simulink library "VIS_TMS_LIB"  (Simulink 8.8)
settings: Solver=VariableStepAuto  StartTime=0.0  StopTime=10.0  RelTol=1e-3  EnableMultiTasking=on
libraries: cdsEpicsOut x50, cdsFilt x39, cdsFiltCtrl x26, cdsTP x24, cdsEpicsIn x15, cdsRms x12, cdsMuxMatrix x6, cdsEpicsStringIn x6, cdsBit2Word x4, cdsEpicsBinIn x4, cdsWord2Bit x2, VIS_LIB x2
(part 1 of 7)
settings Model: SuppressorTable=22 serialization::archive 11 0 3 0 0 0 11 0  Creator=controls  LastModifiedBy=controls

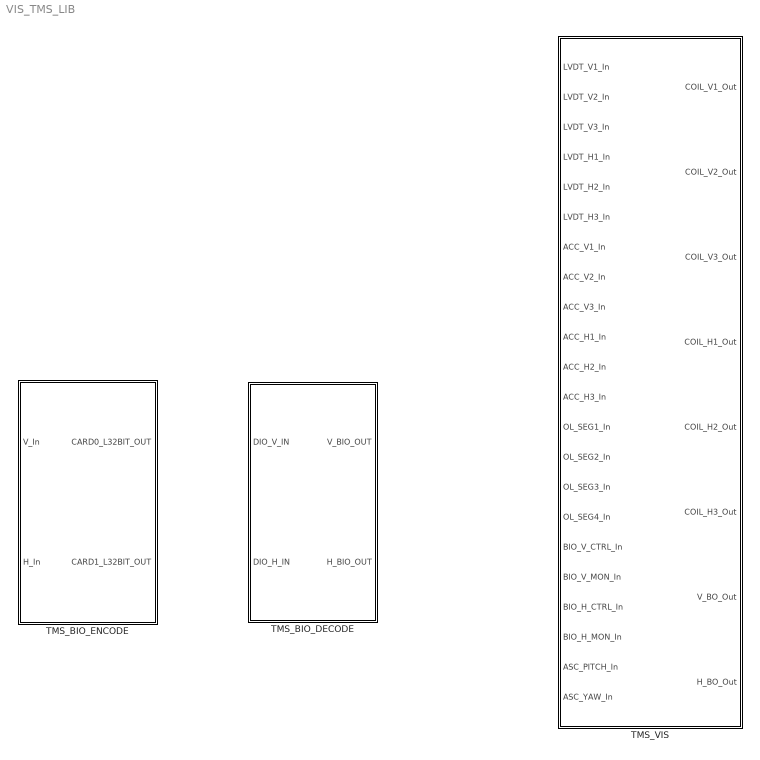
== system VIS_TMS_LIB ==
  TMS_BIO_DECODE : Subsystem
  TMS_BIO_ENCODE : Subsystem
  TMS_VIS : Subsystem

== system VIS_TMS_LIB/TMS_BIO_DECODE ==
  DIO_V_IN : Inport
  DIO_H_IN : Inport  Port=2
  BI1_MON : cdsEpicsOut/Subsystem  Tag=cdsEpicsOutput  Description=|
      | Purpose:                                          
      | Output a FE signal to an EPICS channel.           
      |                                                   
      | Operation:                                        
      | Takes input value and passes it to EPICS record.  
      |                                                   
      | Usage:                                            
      | Name the part with the desired EPICS rrecord name.
      settings: AttributesFormatString=%<Tag>
  BI2_MON : cdsEpicsOut/Subsystem  Tag=cdsEpicsOutput  Description=|
      | Purpose:                                          
      | Output a FE signal to an EPICS channel.           
      |                                                   
      | Operation:                                        
      | Takes input value and passes it to EPICS record.  
      |                                                   
      | Usage:                                            
      | Name the part with the desired EPICS rrecord name.
      settings: AttributesFormatString=%<Tag>
  V_BIO_OUT : Outport
  H_BIO_OUT : Outport  Port=2
  wires:
  DIO_H_IN/1 -> BI2_MON/1
  DIO_V_IN/1 -> BI1_MON/1
  BI1_MON/1 -> V_BIO_OUT/1
  BI2_MON/1 -> H_BIO_OUT/1

== system VIS_TMS_LIB/TMS_BIO_ENCODE ==
  V_In : Inport
  H_In : Inport  Port=2
  BIT2WORD2 : Subsystem
  BIT2WORD3 : Subsystem
  DIO_0_OUT : cdsEpicsOut/Subsystem  Tag=cdsEpicsOutput  Description=|
      | Purpose:                                          
      | Output a FE signal to an EPICS channel.           
      |                                                   
      | Operation:                                        
      | Takes input value and passes it to EPICS record.  
      |                                                   
      | Usage:                                            
      | Name the part with the desired EPICS rrecord name.
      settings: AttributesFormatString=%<Tag>
  DIO_1_OUT : cdsEpicsOut/Subsystem  Tag=cdsEpicsOutput  Description=|
      | Purpose:                                          
      | Output a FE signal to an EPICS channel.           
      |                                                   
      | Operation:                                        
      | Takes input value and passes it to EPICS record.  
      |                                                   
      | Usage:                                            
      | Name the part with the desired EPICS rrecord name.
      settings: AttributesFormatString=%<Tag>
  Ground{2,26,66..67} (4 alike) : Ground
  H_WD_RSET : cdsEpicsBinIn/Subsystem  Tag=cdsEpicsBinIn  Description=|
      | Purpose:                                                                            
      | Create an EPICS binary (0 or 1) input channel to the FE realtime controls.          
      |                                                                                     
      | Operation:                                                                          
      | Outputs value from an EPICS ai record. Value is binary input (bi Epics record type).
      |                                                                                     
      | Usage:                                                                              
      | Name the part with the desired EPICS channel name.
      settings: AttributesFormatString=%<Tag>
  V_WD_RSET : cdsEpicsBinIn/Subsystem  Tag=cdsEpicsBinIn  Description=|
      | Purpose:                                                                            
      | Create an EPICS binary (0 or 1) input channel to the FE realtime controls.          
      |                                                                                     
      | Operation:                                                                          
      | Outputs value from an EPICS ai record. Value is binary input (bi Epics record type).
      |                                                                                     
      | Usage:                                                                              
      | Name the part with the desired EPICS channel name.
      settings: AttributesFormatString=%<Tag>
  cdsWord2Bit : cdsWord2Bit/cdsWord2Bit  Tag=cdsWord2Bit  Description=Generate 16 0/1 outputs from single 16-bit integer input
      settings: AttributesFormatString=cdsWord2Bit
  cdsWord2Bit1 : cdsWord2Bit/cdsWord2Bit  Tag=cdsWord2Bit  Description=Generate 16 0/1 outputs from single 16-bit integer input
      settings: AttributesFormatString=cdsWord2Bit
  CARD0_L32BIT_OUT : Outport
  CARD1_L32BIT_OUT : Outport  Port=2
  wires:
  Ground2/1 -> BIT2WORD2/20(In20), BIT2WORD2/18(In18), BIT2WORD2/19(In19), BIT2WORD2/21(In21), BIT2WORD2/22(In22), BIT2WORD2/23(In23), BIT2WORD2/24(In24), BIT2WORD2/25(In25), BIT2WORD2/26(In26), BIT2WORD2/28(In28), BIT2WORD2/31(In31), BIT2WORD2/32(In32), BIT2WORD2/30(In30), BIT2WORD2/29(In29), BIT2WORD2/27(In27)
  V_In/1 -> cdsWord2Bit/1
  cdsWord2Bit/4 -> BIT2WORD2/4(In4)
  cdsWord2Bit/5 -> BIT2WORD2/5(In5)
  cdsWord2Bit/3 -> BIT2WORD2/3(In3)
  cdsWord2Bit/2 -> BIT2WORD2/2(In2)
  cdsWord2Bit/6 -> BIT2WORD2/6(In6)
  cdsWord2Bit/1 -> BIT2WORD2/1(In1)
  cdsWord2Bit/7 -> BIT2WORD2/7(In7)
  cdsWord2Bit/8 -> BIT2WORD2/8(In8)
  cdsWord2Bit/9 -> BIT2WORD2/9(In9)
  cdsWord2Bit/10 -> BIT2WORD2/10(In10)
  cdsWord2Bit/11 -> BIT2WORD2/11(In11)
  Ground26/1 -> BIT2WORD3/20(In20), BIT2WORD3/18(In18), BIT2WORD3/19(In19), BIT2WORD3/21(In21), BIT2WORD3/22(In22), BIT2WORD3/23(In23), BIT2WORD3/24(In24), BIT2WORD3/25(In25), BIT2WORD3/26(In26), BIT2WORD3/28(In28), BIT2WORD3/31(In31), BIT2WORD3/32(In32), BIT2WORD3/30(In30), BIT2WORD3/29(In29), BIT2WORD3/27(In27)
  H_In/1 -> cdsWord2Bit1/1
  cdsWord2Bit1/4 -> BIT2WORD3/4(In4)
  cdsWord2Bit1/5 -> BIT2WORD3/5(In5)
  cdsWord2Bit1/3 -> BIT2WORD3/3(In3)
  cdsWord2Bit1/2 -> BIT2WORD3/2(In2)
  cdsWord2Bit1/6 -> BIT2WORD3/6(In6)
  cdsWord2Bit1/1 -> BIT2WORD3/1(In1)
  cdsWord2Bit1/7 -> BIT2WORD3/7(In7)
  cdsWord2Bit1/8 -> BIT2WORD3/8(In8)
  cdsWord2Bit1/9 -> BIT2WORD3/9(In9)
  cdsWord2Bit1/10 -> BIT2WORD3/10(In10)
  cdsWord2Bit1/11 -> BIT2WORD3/11(In11)
  Ground66/1 -> H_WD_RSET/1
  Ground67/1 -> V_WD_RSET/1
  H_WD_RSET/1 -> BIT2WORD2/17(In17)
  V_WD_RSET/1 -> BIT2WORD3/17(In17)
  DIO_0_OUT/1 -> CARD0_L32BIT_OUT/1
  BIT2WORD2/1(Out1) -> DIO_0_OUT/1
  BIT2WORD3/1(Out1) -> DIO_1_OUT/1
  DIO_1_OUT/1 -> CARD1_L32BIT_OUT/1
  cdsWord2Bit/12 -> BIT2WORD2/12(In12)
  cdsWord2Bit/13 -> BIT2WORD2/13(In13)
  cdsWord2Bit/14 -> BIT2WORD2/14(In14)
  cdsWord2Bit/15 -> BIT2WORD2/15(In15)
  cdsWord2Bit/16 -> BIT2WORD2/16(In16)
  cdsWord2Bit1/12 -> BIT2WORD3/12(In12)
  cdsWord2Bit1/16 -> BIT2WORD3/16(In16)
  cdsWord2Bit1/14 -> BIT2WORD3/14(In14)
  cdsWord2Bit1/15 -> BIT2WORD3/15(In15)
  cdsWord2Bit1/13 -> BIT2WORD3/13(In13)

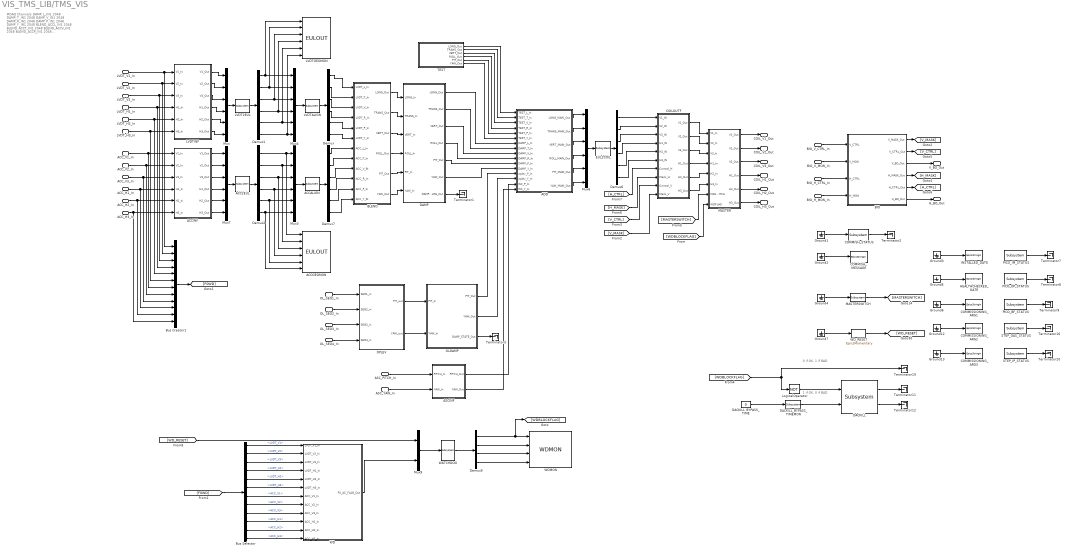
== system VIS_TMS_LIB/TMS_VIS ==
  note: 0 if OK, 1 if BAD
  note: 1 if OK, 0 if BAD
  note: #DAQ Channels
      | DAMP_L_IN1 2048
      | DAMP_T_IN1 2048
      | DAMP_V_IN1 2048
      | DAMP_R_IN1 2048
      | DAMP_P_IN1 2048
      | DAMP_Y_IN1 2048
      | BLEND_ACCL_IN1 2048
      | BLEND_ACCT_IN1 2048
      | BLEND_ACCV_IN1 2048
      | BLEND_ACCR_IN1 2048
      | BLEND_ACCP_IN1 2048
      | BLEND_ACCY_IN1 2048
      | BLEND_LVDTL_IN1 2048
      | BLEND_LVDTT_IN1 2048
      | BLEND_LVDTV_IN1 2048
      | BLEND_LVDTR_IN1 2048
      | BLEND_LVDTP_IN1 2048
      | BLEND_LVDTY_IN1 2048
  LVDT_V1_In : Inport
  LVDT_V2_In : Inport  Port=2
  LVDT_V3_In : Inport  Port=3
  LVDT_H1_In : Inport  Port=4
  LVDT_H2_In : Inport  Port=5
  LVDT_H3_In : Inport  Port=6
  ACC_V1_In : Inport  Port=7
  ACC_V2_In : Inport  Port=8
  ACC_V3_In : Inport  Port=9
  ACC_H1_In : Inport  Port=10
  ACC_H2_In : Inport  Port=11
  ACC_H3_In : Inport  Port=12
  OL_SEG1_In : Inport  Port=13
  OL_SEG2_In : Inport  Port=14
  OL_SEG3_In : Inport  Port=15
  OL_SEG4_In : Inport  Port=16
  BIO_V_CTRL_In : Inport  Port=17
  BIO_V_MON_In : Inport  Port=18
  BIO_H_CTRL_In : Inport  Port=19
  BIO_H_MON_In : Inport  Port=20
  ASC_PITCH_In : Inport  Port=21
  ASC_YAW_In : Inport  Port=22
  ACC2EUL : cdsMuxMatrix/Subsystem  Tag=cdsMuxMatrix  Description=|
      | ADL=SUS_INMATRIX.adl 
      | SCRIPT=generate_KisselButton.py 4 5 #CHANNEL# > #TARGET_DIR#/#FULL_PART_NAME#_KB.adl
      settings: AttributesFormatString=%<Tag>
  ACCALIGN : cdsMuxMatrix/Subsystem  Tag=cdsMuxMatrix  Description=|
      | ADL=SUS_INMATRIX.adl 
      | SCRIPT=generate_KisselButton.py 4 5 #CHANNEL# > #TARGET_DIR#/#FULL_PART_NAME#_KB.adl
      settings: AttributesFormatString=%<Tag>
  ACCGEOMON : VIS_LIB/EULOUT
  ACCINF : Subsystem
  ADD : Subsystem
  ASCINF : Subsystem
  BIO : Subsystem
  BLEND : Subsystem
  Bus Creator1 : BusCreator  Inputs='LVDT_H1','LVDT_H2','LVDT_H3','LVDT_V1','LVDT_V2','LVDT_V3','ACC_H1','ACC_H2','ACC_H3','ACC_V1','ACC_V2','ACC_V3'
  Bus Selector : BusSelector  OutputSignals=LVDT_V1,LVDT_V2,LVDT_V3,LVDT_H1,LVDT_H2,LVDT_H3,ACC_V1,ACC_V2,ACC_V3,ACC_H1,ACC_H2,ACC_H3
  COILOUTF : Subsystem
  COMMISH_MESSAGE : cdsEpicsStringIn/EpicsStringIn  Tag=cdsEpicsStringIn  Description=cdsEpicsStringIn
      settings: AttributesFormatString=%<Tag>
  COMMISH_STATUS : cdsEpicsBinIn/Subsystem  Tag=cdsEpicsBinIn  Description=|
      | Purpose:                                                                            
      | Create an EPICS binary (0 or 1) input channel to the FE realtime controls.          
      |                                                                                     
      | Operation:                                                                          
      | Outputs value from an EPICS ai record. Value is binary input (bi Epics record type).
      |                                                                                     
      | Usage:                                                                              
      | Name the part with the desired EPICS channel name.
      settings: AttributesFormatString=%<Tag>
  COMMISSIONING_ARG1 : cdsEpicsStringIn/EpicsStringIn  Tag=cdsEpicsStringIn  Description=cdsEpicsStringIn
      settings: AttributesFormatString=%<Tag>
  COMMISSIONING_ARG2 : cdsEpicsStringIn/EpicsStringIn  Tag=cdsEpicsStringIn  Description=cdsEpicsStringIn
      settings: AttributesFormatString=%<Tag>
  COMMISSIONING_ARG3 : cdsEpicsStringIn/EpicsStringIn  Tag=cdsEpicsStringIn  Description=cdsEpicsStringIn
      settings: AttributesFormatString=%<Tag>
  DACKILL : cdsDacKill/Subsystem  Description=cdsDacKill
      settings: AttributesFormatString=%<Description>
  DACKILL_BYPASS_TIME : Constant  Value=0
  DACKILL_BYPASS_TIMEMON : cdsEpicsOut/Subsystem  Tag=cdsEpicsOutput  Description=|
      | Purpose:                                          
      | Output a FE signal to an EPICS channel.           
      |                                                   
      | Operation:                                        
      | Takes input value and passes it to EPICS record.  
      |                                                   
      | Usage:                                            
      | Name the part with the desired EPICS rrecord name.
      settings: AttributesFormatString=%<Tag>
  DAMP : Subsystem
  Demux{,1..2,6..7} (5 alike) : Demux  Outputs=6
  Demux9 : Demux
  EUL2COIL : cdsMuxMatrix/Subsystem  Tag=cdsMuxMatrix  Description=|
      | ADL=SUS_INMATRIX.adl 
      | SCRIPT=generate_KisselButton.py 4 5 #CHANNEL# > #TARGET_DIR#/#FULL_PART_NAME#_KB.adl
      settings: AttributesFormatString=%<Tag>
  Ground{1..7,12..13} (9 alike) : Ground
  HEALTHCHECKED_DATE : cdsEpicsStringIn/EpicsStringIn  Tag=cdsEpicsStringIn  Description=cdsEpicsStringIn
      settings: AttributesFormatString=%<Tag>
  INSTALLED_DATE : cdsEpicsStringIn/EpicsStringIn  Tag=cdsEpicsStringIn  Description=cdsEpicsStringIn
      settings: AttributesFormatString=%<Tag>
  LVDT2EUL : cdsMuxMatrix/Subsystem  Tag=cdsMuxMatrix  Description=|
      | ADL=SUS_INMATRIX.adl 
      | SCRIPT=generate_KisselButton.py 4 5 #CHANNEL# > #TARGET_DIR#/#FULL_PART_NAME#_KB.adl
      settings: AttributesFormatString=%<Tag>
  LVDTALIGN : cdsMuxMatrix/Subsystem  Tag=cdsMuxMatrix  Description=|
      | ADL=SUS_INMATRIX.adl 
      | SCRIPT=generate_KisselButton.py 4 5 #CHANNEL# > #TARGET_DIR#/#FULL_PART_NAME#_KB.adl
      settings: AttributesFormatString=%<Tag>
  LVDTGEOMON : VIS_LIB/EULOUT
  LVDTINF : Subsystem
  LogicalOperator : Logic  Operator=NOT  AllPortsSameDT=off  OutDataTypeStr=boolean
  MASTER : Subsystem
  MASTERSWITCH : cdsEpicsBinIn/Subsystem  Tag=cdsEpicsBinIn  Description=|
      | Purpose:                                                                            
      | Create an EPICS binary (0 or 1) input channel to the FE realtime controls.          
      |                                                                                     
      | Operation:                                                                          
      | Outputs value from an EPICS ai record. Value is binary input (bi Epics record type).
      |                                                                                     
      | Usage:                                                                              
      | Name the part with the desired EPICS channel name.
      settings: AttributesFormatString=%<Tag>
  Mux{,3..4,6..7} (5 alike) : Mux  Inputs=6
  Mux9 : Mux  Inputs=2
  OLDAMP : Subsystem
  OPLEV : Subsystem
  PICO_BF_STATUS : cdsEpicsIn/Subsystem  Tag=cdsEpicsIn  Description=|
      | Purpose:                                                                              
      | Create an EPICS input channel connection to the FE realtime controls.                 
      |                                                                                       
      | Operation:                                                                            
      | Outputs value from an EPICS ai record. Value is floating point with a precision of 3..
      |                                                                                       
      | Usage:                                                                                
      | Name the part with the desired EPICS channel name.
      settings: AttributesFormatString=%<Tag>
  PICO_IM_STATUS : cdsEpicsIn/Subsystem  Tag=cdsEpicsIn  Description=|
      | Purpose:                                                                              
      | Create an EPICS input channel connection to the FE realtime controls.                 
      |                                                                                       
      | Operation:                                                                            
      | Outputs value from an EPICS ai record. Value is floating point with a precision of 3..
      |                                                                                       
      | Usage:                                                                                
      | Name the part with the desired EPICS channel name.
      settings: AttributesFormatString=%<Tag>
  PICO_OP_STATUS : cdsEpicsIn/Subsystem  Tag=cdsEpicsIn  Description=|
      | Purpose:                                                                              
      | Create an EPICS input channel connection to the FE realtime controls.                 
      |                                                                                       
      | Operation:                                                                            
      | Outputs value from an EPICS ai record. Value is floating point with a precision of 3..
      |                                                                                       
      | Usage:                                                                                
      | Name the part with the desired EPICS channel name.
      settings: AttributesFormatString=%<Tag>
  STEP_GAS_STATUS : cdsEpicsIn/Subsystem  Tag=cdsEpicsIn  Description=|
      | Purpose:                                                                              
      | Create an EPICS input channel connection to the FE realtime controls.                 
      |                                                                                       
      | Operation:                                                                            
      | Outputs value from an EPICS ai record. Value is floating point with a precision of 3..
      |                                                                                       
      | Usage:                                                                                
      | Name the part with the desired EPICS channel name.
      settings: AttributesFormatString=%<Tag>
  STEP_IP_STATUS : cdsEpicsIn/Subsystem  Tag=cdsEpicsIn  Description=|
      | Purpose:                                                                              
      | Create an EPICS input channel connection to the FE realtime controls.                 
      |                                                                                       
      | Operation:                                                                            
      | Outputs value from an EPICS ai record. Value is floating point with a precision of 3..
      |                                                                                       
      | Usage:                                                                                
      | Name the part with the desired EPICS channel name.
      settings: AttributesFormatString=%<Tag>
  TEST : Subsystem
  Terminator{1..3,7..9,11..12,16,19..20} (11 alike) : Terminator
  WATCHDOG : cdsFunctionCall/Subsystem  Tag=cdsFunctionCall  Description=inline OSEMWATCHDOG /opt/rtcds/userapps/release/vis/common/src/WATCHDOG.c
      settings: AttributesFormatString=%<Tag>\n%<Description>
  WD : Subsystem
  WDMON : SIXOSEM_F_STAGE_MASTER/SIXOSEM_F_STAGE_MASTER/WDMON
  WD_RESET : cdsEpicsMomentary/EpicsMomentary  Tag=cdsEpicsMomentary
      settings: AttributesFormatString=%<Tag>
  COIL_V1_Out : Outport
  COIL_V2_Out : Outport  Port=2
  COIL_V3_Out : Outport  Port=3
  COIL_H1_Out : Outport  Port=4
  COIL_H2_Out : Outport  Port=5
  COIL_H3_Out : Outport  Port=6
  V_BO_Out : Outport  Port=7
  H_BO_Out : Outport  Port=8
  wires:
  MASTER/6(H3_Out) -> COIL_H3_Out/1
  MASTER/5(H2_Out) -> COIL_H2_Out/1
  MASTER/4(H1_Out) -> COIL_H1_Out/1
  MASTER/3(V3_Out) -> COIL_V3_Out/1
  MASTER/2(V2_Out) -> COIL_V2_Out/1
  MASTER/1(V1_Out) -> COIL_V1_Out/1
  COILOUTF/6(H3_Out) -> MASTER/6(H3_In)
  COILOUTF/5(H2_Out) -> MASTER/5(H2_In)
  COILOUTF/4(H1_Out) -> MASTER/4(H1_In)
  COILOUTF/3(V3_Out) -> MASTER/3(V3_In)
  COILOUTF/2(V2_Out) -> MASTER/2(V2_In)
  COILOUTF/1(V1_Out) -> MASTER/1(V1_In)
  Demux6/6 -> COILOUTF/6(H3_IN)
  Demux6/5 -> COILOUTF/5(H2_IN)
  Demux6/4 -> COILOUTF/4(H1_IN)
  Demux6/3 -> COILOUTF/3(V3_IN)
  Demux6/2 -> COILOUTF/2(V2_IN)
  Demux6/1 -> COILOUTF/1(V1_IN)
  Bus Selector/12 -> WD/12(ACC_H3_In)  "<ACC_H3>"
  Bus Selector/11 -> WD/11(ACC_H2_In)  "<ACC_H2>"
  Bus Selector/10 -> WD/10(ACC_H1_In)  "<ACC_H1>"
  Bus Selector/9 -> WD/9(ACC_V3_In)  "<ACC_V3>"
  Bus Selector/8 -> WD/8(ACC_V2_In)  "<ACC_V2>"
  Bus Selector/7 -> WD/7(ACC_V1_In)  "<ACC_V1>"
  Bus Selector/6 -> WD/6(LVDT_H3_In)  "<LVDT_H3>"
  Bus Selector/5 -> WD/5(LVDT_H2_In)  "<LVDT_H2>"
  Bus Selector/4 -> WD/4(LVDT_H1_In)  "<LVDT_H1>"
  Bus Selector/3 -> WD/3(LVDT_V3_In)  "<LVDT_V3>"
  Bus Selector/2 -> WD/2(LVDT_V2_In)  "<LVDT_V2>"
  Bus Selector/1 -> WD/1(LVDT_V1_In)  "<LVDT_V1>"
  ACC_H3_In/1 -> ACCINF/6(H3_In), Bus Creator1/12
  ACC_H2_In/1 -> ACCINF/5(H2_In), Bus Creator1/11
  ACC_H1_In/1 -> ACCINF/4(H1_In), Bus Creator1/10
  ACC_V3_In/1 -> ACCINF/3(V3_In), Bus Creator1/9
  ACC_V2_In/1 -> ACCINF/2(V2_In), Bus Creator1/8
  ACC_V1_In/1 -> ACCINF/1(V1_In), Bus Creator1/7
  LVDT_H3_In/1 -> LVDTINF/6(H3_In), Bus Creator1/6
  LVDT_H2_In/1 -> LVDTINF/5(H2_In), Bus Creator1/5
  LVDT_H1_In/1 -> LVDTINF/4(H1_In), Bus Creator1/4
  LVDT_V3_In/1 -> LVDTINF/3(V3_In), Bus Creator1/3
  LVDT_V2_In/1 -> LVDTINF/2(V2_In), Bus Creator1/2
  LVDT_V1_In/1 -> LVDTINF/1(V1_In), Bus Creator1/1
  ACCINF/6(H3_Out) -> Mux7/6
  ACCINF/5(H2_Out) -> Mux7/5
  ACCINF/4(H1_Out) -> Mux7/4
  ACCINF/3(V3_Out) -> Mux7/3
  ACCINF/2(V2_Out) -> Mux7/2
  ACCINF/1(V1_Out) -> Mux7/1
  LVDTINF/6(H3_Out) -> Mux/6
  LVDTINF/5(H2_Out) -> Mux/5
  LVDTINF/4(H1_Out) -> Mux/4
  LVDTINF/3(V3_Out) -> Mux/3
  LVDTINF/2(V2_Out) -> Mux/2
  LVDTINF/1(V1_Out) -> Mux/1
  OLDAMP/3(DAMP_STATE_Out) -> Terminator3/1
  OLDAMP/2(YAW_Out) -> ADD/14(oplev_Y_In)
  OLDAMP/1(PIT_Out) -> ADD/13(oplev_P_In)
  OPLEV/2(YAW_out) -> OLDAMP/2(YAW_In)
  OPLEV/1(PIT_out) -> OLDAMP/1(PIT_In)
  WD_RESET/1 -> [WD_RESET]
  Ground7/1 -> WD_RESET/1
  Ground4/1 -> MASTERSWITCH/1
  MASTERSWITCH/1 -> [MASTERSWITCH]
  Ground2/1 -> COMMISH_MESSAGE/1
  COMMISH_STATUS/1 -> Terminator2/1
  Ground1/1 -> COMMISH_STATUS/1
  [WDBLOCKFLAG] -> Terminator19/1, LogicalOperator/1
  LogicalOperator/1 -> DACKILL/1
  DACKILL_BYPASS_TIMEMON/1 -> DACKILL/2
  DACKILL_BYPASS_TIME/1 -> DACKILL_BYPASS_TIMEMON/1
  DACKILL/1 -> Terminator11/1
  DACKILL/2 -> Terminator12/1
  BIO_H_MON_In/1 -> BIO/4(H_MON)
  BIO_H_CTRL_In/1 -> BIO/3(H_CTRL)
  BIO_V_MON_In/1 -> BIO/2(V_MON)
  BIO_V_CTRL_In/1 -> BIO/1(V_CTRL)
  [V_MASK] -> COILOUTF/10(Mask_V)
  [V_CTRL] -> COILOUTF/9(Control_V)
  [H_MASK] -> COILOUTF/8(Mask_H)
  [H_CTRL] -> COILOUTF/7(Control_H)
  BIO/6(H_BO_Out) -> H_BO_Out/1
  BIO/3(V_BO_Out) -> V_BO_Out/1
  BIO/5(H_CTRL_Out) -> [H_CTRL]
  BIO/2(V_CTRL_Out) -> [V_CTRL]
  BIO/4(H_MASK_Out) -> [H_MASK]
  BIO/1(V_MASK_Out) -> [V_MASK]
  OL_SEG4_In/1 -> OPLEV/4(SEG4_in)
  OL_SEG3_In/1 -> OPLEV/3(SEG3_in)
  OL_SEG2_In/1 -> OPLEV/2(SEG2_in)
  OL_SEG1_In/1 -> OPLEV/1(SEG1_in)
  ADD/6(YAW_MAIN_Out) -> Mux6/6
  ADD/5(PIT_MAIN_Out) -> Mux6/5
  ADD/4(ROLL_MAIN_Out) -> Mux6/4
  ADD/3(VERT_MAIN_Out) -> Mux6/3
  ADD/2(TRANS_MAIN_Out) -> Mux6/2
  ADD/1(LONG_MAIN_Out) -> Mux6/1
  TEST/6(YAW_Out) -> ADD/6(TEST_Y_In)
  TEST/5(PIT_Out) -> ADD/5(TEST_P_In)
  TEST/4(ROLL_Out) -> ADD/4(TEST_R_In)
  DAMP/6(YAW_Out) -> ADD/12(DAMP_Y_In)
  DAMP/5(PIT_Out) -> ADD/11(DAMP_P_In)
  DAMP/4(ROLL_Out) -> ADD/10(DAMP_R_In)
  BLEND/6(YAW_Out) -> DAMP/6(YAW_In)
  BLEND/5(PIT_Out) -> DAMP/5(PIT_In)
  BLEND/4(ROLL_Out) -> DAMP/4(ROLL_In)
  BLEND/3(VERT_Out) -> DAMP/3(VERT_In)
  BLEND/2(TRANS_Out) -> DAMP/2(TRANS_In)
  BLEND/1(LONG_Out) -> DAMP/1(LONG_In)
  Demux7/1 -> BLEND/7(ACC_L_In)
  Demux7/2 -> BLEND/8(ACC_T_In)
  Demux7/3 -> BLEND/9(ACC_V_IN)
  Demux7/4 -> BLEND/10(ACC_R_In)
  Demux7/5 -> BLEND/11(ACC_P_In)
  Demux7/6 -> BLEND/12(ACC_Y_IN)
  Demux/4 -> BLEND/4(LVDT_R_In)
  Mux/1 -> LVDT2EUL/1
  LVDT2EUL/1 -> Demux1/1
  ACCALIGN/1 -> Demux7/1
  Demux/1 -> BLEND/1(LVDT_L_In)
  Demux/2 -> BLEND/2(LVDT_T_In)
  Demux/3 -> BLEND/3(LVDT_V_In)
  Mux6/1 -> EUL2COIL/1
  EUL2COIL/1 -> Demux6/1
  [MASTERSWITCH] -> MASTER/7(MASTERSWITCH)
  [WD_RESET] -> Mux9/1
  WD/1(F0_AC_FLAG_Out) -> Mux9/2
  [F0WD] -> Bus Selector/1
  Demux9/1 -> [WDBLOCKFLAG], WDMON/1
  Demux9/2 -> WDMON/2
  Demux9/3 -> WDMON/3
  Demux9/4 -> WDMON/4
  Mux9/1 -> WATCHDOG/1
  WATCHDOG/1 -> Demux9/1
  Bus Creator1/1 -> [F0WD]
  [WDBLOCKFLAG] -> MASTER/8(WDFLAG)
  DAMP/7(DAMP_STATE_Out) -> Terminator1/1
  TEST/1(LONG_Out) -> ADD/1(TEST_L_In)
  TEST/2(TRANS_Out) -> ADD/2(TEST_T_In)
  TEST/3(VERT_Out) -> ADD/3(TEST_V_In)
  DAMP/1(LONG_Out) -> ADD/7(DAMP_L_In)
  DAMP/2(TRANS_Out) -> ADD/8(DAMP_T_In)
  DAMP/3(VERT_Out) -> ADD/9(DAMP_V_In)
  ASC_PITCH_In/1 -> ASCINF/1(PITCH_In)
  ASC_YAW_In/1 -> ASCINF/2(YAW_In)
  ASCINF/1(PITCH_Out) -> ADD/15(ISC_P_In)
  ASCINF/2(YAW_Out) -> ADD/16(ISC_Y_In)
  Demux/5 -> BLEND/5(LVDT_P_In)
  Demux/6 -> BLEND/6(LVDT_Y_In)
  Mux4/1 -> LVDTALIGN/1
  LVDTALIGN/1 -> Demux/1
  Mux3/1 -> ACCALIGN/1
  Mux7/1 -> ACC2EUL/1
  ACC2EUL/1 -> Demux2/1
  Demux1/1 -> LVDTGEOMON/1, Mux4/1
  Demux1/2 -> LVDTGEOMON/2, Mux4/2
  Demux1/3 -> LVDTGEOMON/3, Mux4/3
  Demux1/4 -> LVDTGEOMON/4, Mux4/4
  Demux1/5 -> LVDTGEOMON/5, Mux4/5
  Demux1/6 -> LVDTGEOMON/6, Mux4/6
  Demux2/2 -> ACCGEOMON/2, Mux3/2
  Demux2/3 -> ACCGEOMON/3, Mux3/3
  Demux2/4 -> ACCGEOMON/4, Mux3/4
  Demux2/5 -> ACCGEOMON/5, Mux3/5
  Demux2/6 -> ACCGEOMON/6, Mux3/6
  Demux2/1 -> ACCGEOMON/1, Mux3/1
  Ground3/1 -> INSTALLED_DATE/1
  Ground5/1 -> HEALTHCHECKED_DATE/1
  STEP_IP_STATUS/1 -> Terminator20/1
  STEP_GAS_STATUS/1 -> Terminator16/1
  PICO_BF_STATUS/1 -> Terminator9/1
  PICO_IM_STATUS/1 -> Terminator7/1
  PICO_OP_STATUS/1 -> Terminator8/1
  Ground6/1 -> COMMISSIONING_ARG1/1
  Ground12/1 -> COMMISSIONING_ARG2/1
  Ground13/1 -> COMMISSIONING_ARG3/1

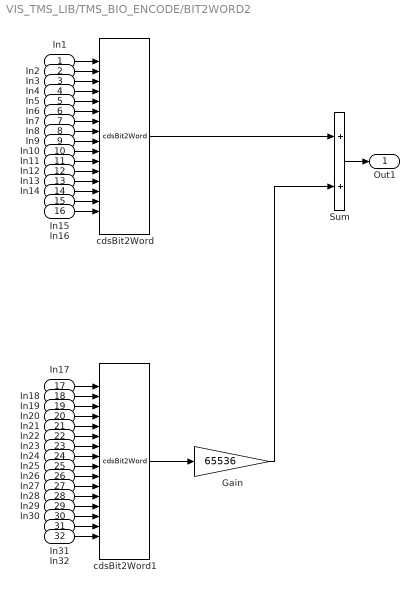
== system VIS_TMS_LIB/TMS_BIO_ENCODE/BIT2WORD2 ==
  In1 : Inport
  In2 : Inport  Port=2
  In3 : Inport  Port=3
  In4 : Inport  Port=4
  In5 : Inport  Port=5
  In6 : Inport  Port=6
  In7 : Inport  Port=7
  In8 : Inport  Port=8
  In9 : Inport  Port=9
  In10 : Inport  Port=10
  In11 : Inport  Port=11
  In12 : Inport  Port=12
  In13 : Inport  Port=13
  In14 : Inport  Port=14
  In15 : Inport  Port=15
  In16 : Inport  Port=16
  In17 : Inport  Port=17
  In18 : Inport  Port=18
  In19 : Inport  Port=19
  In20 : Inport  Port=20
  In21 : Inport  Port=21
  In22 : Inport  Port=22
  In23 : Inport  Port=23
  In24 : Inport  Port=24
  In25 : Inport  Port=25
  In26 : Inport  Port=26
  In27 : Inport  Port=27
  In28 : Inport  Port=28
  In29 : Inport  Port=29
  In30 : Inport  Port=30
  In31 : Inport  Port=31
  In32 : Inport  Port=32
  Gain : Gain  Gain=65536
  Sum : Sum
  cdsBit2Word : cdsBit2Word/cdsBit2Word  Tag=cdsBit2Word  Description=Forms single 16 bit integer from 16 0/1 inputs.
      settings: AttributesFormatString=%<Tag>
  cdsBit2Word1 : cdsBit2Word/cdsBit2Word  Tag=cdsBit2Word  Description=Forms single 16 bit integer from 16 0/1 inputs.
      settings: AttributesFormatString=%<Tag>
  Out1 : Outport
  wires:
  Gain/1 -> Sum/2
  cdsBit2Word1/1 -> Gain/1
  cdsBit2Word/1 -> Sum/1
  In1/1 -> cdsBit2Word/1
  In2/1 -> cdsBit2Word/2
  In3/1 -> cdsBit2Word/3
  In4/1 -> cdsBit2Word/4
  In5/1 -> cdsBit2Word/5
  In6/1 -> cdsBit2Word/6
  In7/1 -> cdsBit2Word/7
  In8/1 -> cdsBit2Word/8
  In9/1 -> cdsBit2Word/9
  In10/1 -> cdsBit2Word/10
  Sum/1 -> Out1/1
  In11/1 -> cdsBit2Word/11
  In12/1 -> cdsBit2Word/12
  In13/1 -> cdsBit2Word/13
  In14/1 -> cdsBit2Word/14
  In15/1 -> cdsBit2Word/15
  In16/1 -> cdsBit2Word/16
  In17/1 -> cdsBit2Word1/1
  In18/1 -> cdsBit2Word1/2
  In19/1 -> cdsBit2Word1/3
  In20/1 -> cdsBit2Word1/4
  In21/1 -> cdsBit2Word1/5
  In22/1 -> cdsBit2Word1/6
  In23/1 -> cdsBit2Word1/7
  In24/1 -> cdsBit2Word1/8
  In25/1 -> cdsBit2Word1/9
  In26/1 -> cdsBit2Word1/10
  In27/1 -> cdsBit2Word1/11
  In28/1 -> cdsBit2Word1/12
  In29/1 -> cdsBit2Word1/13
  In30/1 -> cdsBit2Word1/14
  In31/1 -> cdsBit2Word1/15
  In32/1 -> cdsBit2Word1/16

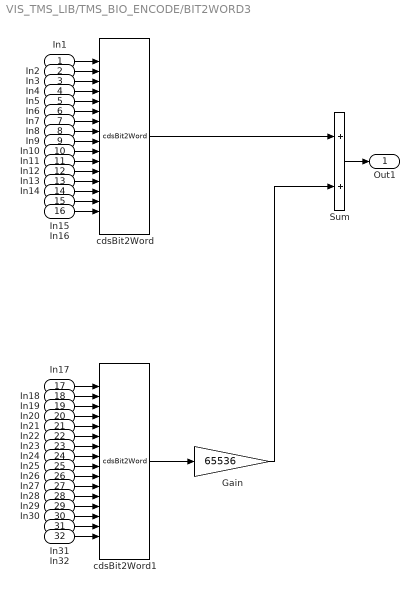
== system VIS_TMS_LIB/TMS_BIO_ENCODE/BIT2WORD3 ==
  In1 : Inport
  In2 : Inport  Port=2
  In3 : Inport  Port=3
  In4 : Inport  Port=4
  In5 : Inport  Port=5
  In6 : Inport  Port=6
  In7 : Inport  Port=7
  In8 : Inport  Port=8
  In9 : Inport  Port=9
  In10 : Inport  Port=10
  In11 : Inport  Port=11
  In12 : Inport  Port=12
  In13 : Inport  Port=13
  In14 : Inport  Port=14
  In15 : Inport  Port=15
  In16 : Inport  Port=16
  In17 : Inport  Port=17
  In18 : Inport  Port=18
  In19 : Inport  Port=19
  In20 : Inport  Port=20
  In21 : Inport  Port=21
  In22 : Inport  Port=22
  In23 : Inport  Port=23
  In24 : Inport  Port=24
  In25 : Inport  Port=25
  In26 : Inport  Port=26
  In27 : Inport  Port=27
  In28 : Inport  Port=28
  In29 : Inport  Port=29
  In30 : Inport  Port=30
  In31 : Inport  Port=31
  In32 : Inport  Port=32
  Gain : Gain  Gain=65536
  Sum : Sum
  cdsBit2Word : cdsBit2Word/cdsBit2Word  Tag=cdsBit2Word  Description=Forms single 16 bit integer from 16 0/1 inputs.
      settings: AttributesFormatString=%<Tag>
  cdsBit2Word1 : cdsBit2Word/cdsBit2Word  Tag=cdsBit2Word  Description=Forms single 16 bit integer from 16 0/1 inputs.
      settings: AttributesFormatString=%<Tag>
  Out1 : Outport
  wires:
  Gain/1 -> Sum/2
  cdsBit2Word1/1 -> Gain/1
  cdsBit2Word/1 -> Sum/1
  In1/1 -> cdsBit2Word/1
  In2/1 -> cdsBit2Word/2
  In3/1 -> cdsBit2Word/3
  In4/1 -> cdsBit2Word/4
  In5/1 -> cdsBit2Word/5
  In6/1 -> cdsBit2Word/6
  In7/1 -> cdsBit2Word/7
  In8/1 -> cdsBit2Word/8
  In9/1 -> cdsBit2Word/9
  In10/1 -> cdsBit2Word/10
  Sum/1 -> Out1/1
  In11/1 -> cdsBit2Word/11
  In12/1 -> cdsBit2Word/12
  In13/1 -> cdsBit2Word/13
  In14/1 -> cdsBit2Word/14
  In15/1 -> cdsBit2Word/15
  In16/1 -> cdsBit2Word/16
  In17/1 -> cdsBit2Word1/1
  In18/1 -> cdsBit2Word1/2
  In19/1 -> cdsBit2Word1/3
  In20/1 -> cdsBit2Word1/4
  In21/1 -> cdsBit2Word1/5
  In22/1 -> cdsBit2Word1/6
  In23/1 -> cdsBit2Word1/7
  In24/1 -> cdsBit2Word1/8
  In25/1 -> cdsBit2Word1/9
  In26/1 -> cdsBit2Word1/10
  In27/1 -> cdsBit2Word1/11
  In28/1 -> cdsBit2Word1/12
  In29/1 -> cdsBit2Word1/13
  In30/1 -> cdsBit2Word1/14
  In31/1 -> cdsBit2Word1/15
  In32/1 -> cdsBit2Word1/16

== system VIS_TMS_LIB/TMS_VIS/ACCINF ==
  V1_In : Inport
  V2_In : Inport  Port=2
  V3_In : Inport  Port=3
  H1_In : Inport  Port=4
  H2_In : Inport  Port=5
  H3_In : Inport  Port=6
  H1 : cdsFilt/Subsystem  Tag=cdsFilt  Description=|
      | Purpose:                                                                                                                                                                                                                                  
      | Standard CDS IIR filter module.                                                                                                                                                                                                           
      |                                                                                                                                                                                                                                           
      | Operation:                                                                                                                                                                                                                                
      | Consists of 10 second order section IIR filters, plus a ramped gain stage. In FE code, also provides pre-defined test points and excitation channel inputs. The filter coefficients are defined in the LIGO system using the 'foton' tool.
      |                                                                                                                                                                                                                                           
      | Usage:                                                                                                                                                                                                                                    
      | Name the part with the desired filter module name.
      settings: AttributesFormatString=%<Tag>
  H2 : cdsFilt/Subsystem  Tag=cdsFilt  Description=|
      | Purpose:                                                                                                                                                                                                                                  
      | Standard CDS IIR filter module.                                                                                                                                                                                                           
      |                                                                                                                                                                                                                                           
      | Operation:                                                                                                                                                                                                                                
      | Consists of 10 second order section IIR filters, plus a ramped gain stage. In FE code, also provides pre-defined test points and excitation channel inputs. The filter coefficients are defined in the LIGO system using the 'foton' tool.
      |                                                                                                                                                                                                                                           
      | Usage:                                                                                                                                                                                                                                    
      | Name the part with the desired filter module name.
      settings: AttributesFormatString=%<Tag>
  H3 : cdsFilt/Subsystem  Tag=cdsFilt  Description=|
      | Purpose:                                                                                                                                                                                                                                  
      | Standard CDS IIR filter module.                                                                                                                                                                                                           
      |                                                                                                                                                                                                                                           
      | Operation:                                                                                                                                                                                                                                
      | Consists of 10 second order section IIR filters, plus a ramped gain stage. In FE code, also provides pre-defined test points and excitation channel inputs. The filter coefficients are defined in the LIGO system using the 'foton' tool.
      |                                                                                                                                                                                                                                           
      | Usage:                                                                                                                                                                                                                                    
      | Name the part with the desired filter module name.
      settings: AttributesFormatString=%<Tag>
  V1 : cdsFilt/Subsystem  Tag=cdsFilt  Description=|
      | Purpose:                                                                                                                                                                                                                                  
      | Standard CDS IIR filter module.                                                                                                                                                                                                           
      |                                                                                                                                                                                                                                           
      | Operation:                                                                                                                                                                                                                                
      | Consists of 10 second order section IIR filters, plus a ramped gain stage. In FE code, also provides pre-defined test points and excitation channel inputs. The filter coefficients are defined in the LIGO system using the 'foton' tool.
      |                                                                                                                                                                                                                                           
      | Usage:                                                                                                                                                                                                                                    
      | Name the part with the desired filter module name.
      settings: AttributesFormatString=%<Tag>
  V2 : cdsFilt/Subsystem  Tag=cdsFilt  Description=|
      | Purpose:                                                                                                                                                                                                                                  
      | Standard CDS IIR filter module.                                                                                                                                                                                                           
      |                                                                                                                                                                                                                                           
      | Operation:                                                                                                                                                                                                                                
      | Consists of 10 second order section IIR filters, plus a ramped gain stage. In FE code, also provides pre-defined test points and excitation channel inputs. The filter coefficients are defined in the LIGO system using the 'foton' tool.
      |                                                                                                                                                                                                                                           
      | Usage:                                                                                                                                                                                                                                    
      | Name the part with the desired filter module name.
      settings: AttributesFormatString=%<Tag>
  V3 : cdsFilt/Subsystem  Tag=cdsFilt  Description=|
      | Purpose:                                                                                                                                                                                                                                  
      | Standard CDS IIR filter module.                                                                                                                                                                                                           
      |                                                                                                                                                                                                                                           
      | Operation:                                                                                                                                                                                                                                
      | Consists of 10 second order section IIR filters, plus a ramped gain stage. In FE code, also provides pre-defined test points and excitation channel inputs. The filter coefficients are defined in the LIGO system using the 'foton' tool.
      |                                                                                                                                                                                                                                           
      | Usage:                                                                                                                                                                                                                                    
      | Name the part with the desired filter module name.
      settings: AttributesFormatString=%<Tag>
  V1_Out : Outport
  V2_Out : Outport  Port=2
  V3_Out : Outport  Port=3
  H1_Out : Outport  Port=4
  H2_Out : Outport  Port=5
  H3_Out : Outport  Port=6
  wires:
  V1_In/1 -> V1/1
  V1/1 -> V1_Out/1
  V2_In/1 -> V2/1
  V2/1 -> V2_Out/1
  V3_In/1 -> V3/1
  V3/1 -> V3_Out/1
  H1_In/1 -> H1/1
  H1/1 -> H1_Out/1
  H2_In/1 -> H2/1
  H2/1 -> H2_Out/1
  H3_In/1 -> H3/1
  H3/1 -> H3_Out/1

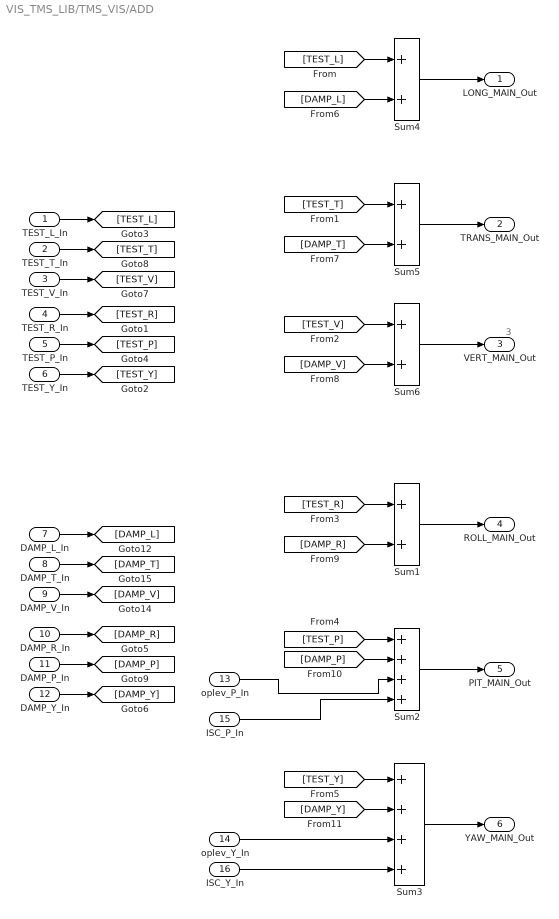
== system VIS_TMS_LIB/TMS_VIS/ADD ==
  note: 3
  TEST_L_In : Inport
  TEST_T_In : Inport  Port=2
  TEST_V_In : Inport  Port=3
  TEST_R_In : Inport  Port=4
  TEST_P_In : Inport  Port=5
  TEST_Y_In : Inport  Port=6
  DAMP_L_In : Inport  Port=7
  DAMP_T_In : Inport  Port=8
  DAMP_V_In : Inport  Port=9
  DAMP_R_In : Inport  Port=10
  DAMP_P_In : Inport  Port=11
  DAMP_Y_In : Inport  Port=12
  oplev_P_In : Inport  Port=13
  oplev_Y_In : Inport  Port=14
  ISC_P_In : Inport  Port=15
  ISC_Y_In : Inport  Port=16
  Sum{1,4..6} (4 alike) : Sum
  Sum2 : Sum  Inputs=++++
  Sum3 : Sum  Inputs=++++
  LONG_MAIN_Out : Outport
  TRANS_MAIN_Out : Outport  Port=2
  VERT_MAIN_Out : Outport  Port=3
  ROLL_MAIN_Out : Outport  Port=4
  PIT_MAIN_Out : Outport  Port=5
  YAW_MAIN_Out : Outport  Port=6
  wires:
  oplev_P_In/1 -> Sum2/3
  [DAMP_Y] -> Sum3/2
  [DAMP_P] -> Sum2/2
  [DAMP_R] -> Sum1/2
  [DAMP_V] -> Sum6/2
  [DAMP_T] -> Sum5/2
  [DAMP_L] -> Sum4/2
  [TEST_Y] -> Sum3/1
  [TEST_P] -> Sum2/1
  [TEST_R] -> Sum1/1
  [TEST_V] -> Sum6/1
  [TEST_T] -> Sum5/1
  [TEST_L] -> Sum4/1
  DAMP_R_In/1 -> [DAMP_R]
  DAMP_P_In/1 -> [DAMP_P]
  DAMP_Y_In/1 -> [DAMP_Y]
  Sum6/1 -> VERT_MAIN_Out/1
  Sum4/1 -> LONG_MAIN_Out/1
  Sum5/1 -> TRANS_MAIN_Out/1
  TEST_R_In/1 -> [TEST_R]
  TEST_P_In/1 -> [TEST_P]
  TEST_Y_In/1 -> [TEST_Y]
  Sum1/1 -> ROLL_MAIN_Out/1
  TEST_L_In/1 -> [TEST_L]
  TEST_T_In/1 -> [TEST_T]
  TEST_V_In/1 -> [TEST_V]
  DAMP_L_In/1 -> [DAMP_L]
  DAMP_T_In/1 -> [DAMP_T]
  DAMP_V_In/1 -> [DAMP_V]
  Sum2/1 -> PIT_MAIN_Out/1
  Sum3/1 -> YAW_MAIN_Out/1
  oplev_Y_In/1 -> Sum3/3
  ISC_P_In/1 -> Sum2/4
  ISC_Y_In/1 -> Sum3/4

== system VIS_TMS_LIB/TMS_VIS/ASCINF ==
  PITCH_In : Inport
  YAW_In : Inport  Port=2
  P : cdsFilt/Subsystem  Tag=cdsFilt  Description=|
      | Purpose:                                                                                                                                                                                                                                  
      | Standard CDS IIR filter module.                                                                                                                                                                                                           
      |                                                                                                                                                                                                                                           
      | Operation:                                                                                                                                                                                                                                
      | Consists of 10 second order section IIR filters, plus a ramped gain stage. In FE code, also provides pre-defined test points and excitation channel inputs. The filter coefficients are defined in the LIGO system using the 'foton' tool.
      |                                                                                                                                                                                                                                           
      | Usage:                                                                                                                                                                                                                                    
      | Name the part with the desired filter module name.
      settings: AttributesFormatString=%<Tag>
  Y : cdsFilt/Subsystem  Tag=cdsFilt  Description=|
      | Purpose:                                                                                                                                                                                                                                  
      | Standard CDS IIR filter module.                                                                                                                                                                                                           
      |                                                                                                                                                                                                                                           
      | Operation:                                                                                                                                                                                                                                
      | Consists of 10 second order section IIR filters, plus a ramped gain stage. In FE code, also provides pre-defined test points and excitation channel inputs. The filter coefficients are defined in the LIGO system using the 'foton' tool.
      |                                                                                                                                                                                                                                           
      | Usage:                                                                                                                                                                                                                                    
      | Name the part with the desired filter module name.
      settings: AttributesFormatString=%<Tag>
  PITCH_Out : Outport
  YAW_Out : Outport  Port=2
  wires:
  PITCH_In/1 -> P/1
  YAW_In/1 -> Y/1
  P/1 -> PITCH_Out/1
  Y/1 -> YAW_Out/1

== system VIS_TMS_LIB/TMS_VIS/BIO ==
  V_CTRL : Inport
  V_MON : Inport  Port=2
  H_CTRL : Inport  Port=3
  H_MON : Inport  Port=4
  H : STATE_BIO_MASTER/UIM_BIO_MASTER
  V : STATE_BIO_MASTER/UIM_BIO_MASTER
  V_MASK_Out : Outport
  V_CTRL_Out : Outport  Port=2
  V_BO_Out : Outport  Port=3
  H_MASK_Out : Outport  Port=4
  H_CTRL_Out : Outport  Port=5
  H_BO_Out : Outport  Port=6
  wires:
  V/3 -> V_BO_Out/1
  V_MON/1 -> V/2
  V/2 -> V_CTRL_Out/1
  V_CTRL/1 -> V/1
  H/3 -> H_BO_Out/1
  H_CTRL/1 -> H/1
  H_MON/1 -> H/2
  V/1 -> V_MASK_Out/1
  H/1 -> H_MASK_Out/1
  H/2 -> H_CTRL_Out/1
